simulink model "BasicPumpPlant"  (R2022b)
settings: Solver=VariableStepAuto  StartTime=0.0  StopTime=10.0  RelTol=1e-3
values from neighbouring files (symbols this model uses):
  AN403992StandardFlowMotorMaxDisp_ccperrev = 9.8*2.1    (= 20.58)    [Cascade_SolutionPumpModel_DD.m]
  MotorPumpDampingCoef = 2.630416384778607e-04    (= 0.000263041638478)    [Cascade_SolutionPumpModel_DD.m]
  Pascal_To_psi = 0.0001450377    [Cascade_SolutionPumpModel_DD.m]
undefined symbols (not defined in the file or in its folder): AN402280HighFlowPumpBrakePowerNQ2D_HP, AN403993HighFlowMotorMaxDisp_ccperrev
libraries: fl_lib x21, nesl_utility x9, sh_lib x8, fl_ps_legacy_lib x6, slpidlib x1
settings Model: Creator=pm16590  LastModifiedBy=tilog
settings DataIOCC: ReturnWorkspaceOutputs=off
settings DebuggingCC: UnconnectedInputMsg=warning  UnconnectedOutputMsg=warning  UnconnectedLineMsg=warning  SFMachineParentedDataDiag=warning  ArithmeticOperatorsInVariantConditions=warning
settings ModelReferenceCC: EnableRefExpFcnMdlSchedulingChecks=on
settings SFSimCC: CustomCodeUndefinedFunction=UseInterfaceOnly

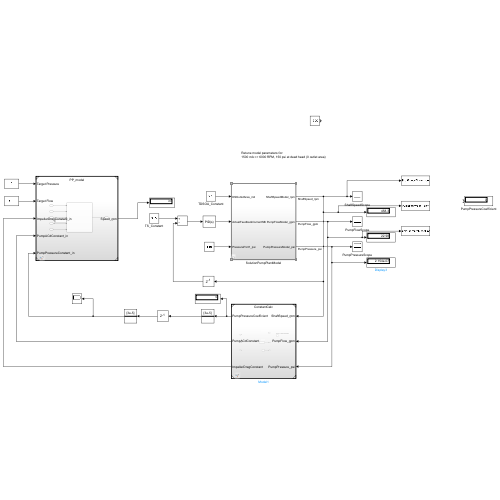
[thumbnail: Simulink's stored preview of the top-level diagram]
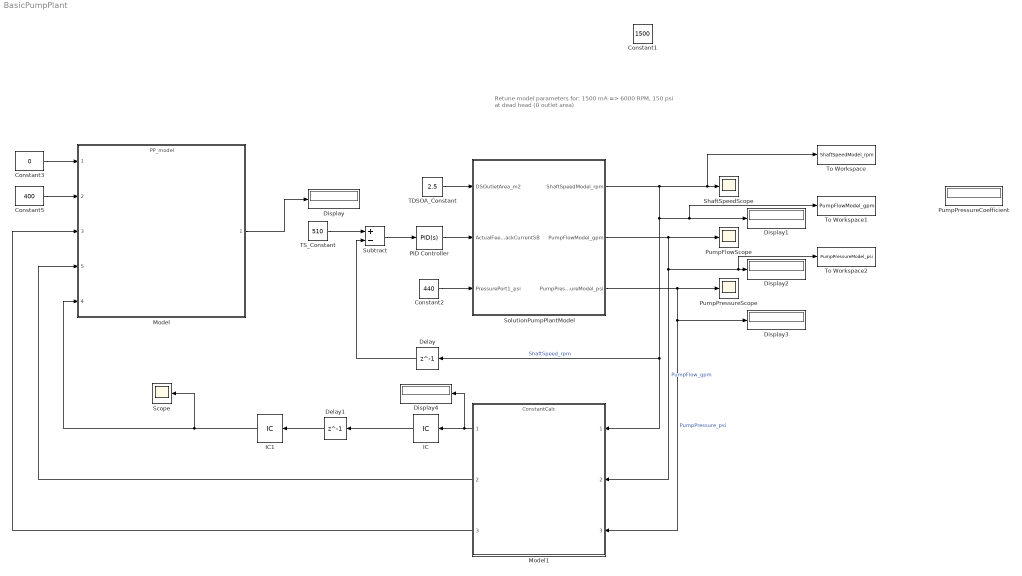
== system BasicPumpPlant ==
  note: Retune model parameters for:
      | 1500 mA => 6000 RPM, 150 psi at dead head (0 outlet area)
  Constant1 : Constant  Value=1500
  Constant2 : Constant  Value=440
  Constant3 : Constant  Value=0
  Constant5 : Constant  Value=400
  Delay : Delay  DelayLength=1  InitialCondition=1
  Delay1 : Delay  DelayLength=1  InitialCondition=1
  Display{,1..4} (5 alike) : Display
  IC : InitialCondition  Value=3e-5
  IC1 : InitialCondition  Value=3e-5
  Model : ModelReference  ModelNameDialog=PP_model.slx  SimulationMode=Normal  ModelReferenceVersion=1.5
      settings: PortSchema="{\"entries\":[{\"content\":{\"sides\":[{\"content\":{\"connectorIds\":[\"In1\",\"In2\",\"In3\",\"In5\",\"In4\"]},\"type\":\"ConnectorPlacement.EquallySpacedRectSide\",\"uuid\":\"fdcef34a-74c4-4aee-b0bc-6e3e5f9e7ac2\"},{\"content\":{\"connectorIds\":[\"Out1\"],\"side\":\"RIGHT\"},\"type\":\"ConnectorPlacement.EquallySpacedRectSide\",\"uuid\":\"cb4b70af-0550-4c5a-8289-d3aa2bf45742\"},{\"content\":{\"connectorIds\":[],\"side\":\"TOP\"},\"type\":\"ConnectorPlacement.EquallySpacedRectSide\",\"uuid\":\"87759187-0da6-406f-b9db-6c95d92bffe7\"}]},\"type\":\"ConnectorPlacement.EquallySpacedConnector\",\"uuid\":\"123e04ed-575d-4795-8cdc-174c34b6de50\"}],\"packageUris\":[\"http://schema.mathworks.com/mf0/Connector/R2020b\"],\"version\":\"1.0\"}"
  Model1 : ModelReference  ModelNameDialog=ConstantCalc.slx  SimulationMode=Normal  ModelReferenceVersion=1.11
  PID Controller : slpidlib/PID Controller  Controller=PID  Form=Parallel  TimeDomain=Continuous-time  UseExternalTs=off  SampleTime=-1  IntegratorMethod=Forward Euler  FilterMethod=Forward Euler  ControllerParametersSource=internal  P=0  I=.1  UseKiTs=off  D=0  N=100  UseFilter=on  TunerSelectOption=Transfer Function Based (PID Tuner App)  InitialConditionSource=internal  InitialConditionForIntegrator=0  InitialConditionForFilter=0  DifferentiatorICPrevScaledInput=0  ExternalReset=none  TrackingMode=off  Kt=1  LimitOutput=off  SatLimitsSource=internal  UpperSaturationLimit=inf  LowerSaturationLimit=-inf  LinearizeAsGain=on  AntiWindupMode=none  Kb=1  LimitIntegrator=off  UpperIntegratorSaturationLimit=inf  LowerIntegratorSaturationLimit=-inf  POutMin=[]  POutMax=[]  IOutMin=[]  IOutMax=[]  DOutMin=[]  DOutMax=[]  NOutMin=[]  NOutMax=[]  SumOutMin=[]  SumOutMax=[]  SaturationOutMin=[]  SaturationOutMax=[]  PParamMin=[]  PParamMax=[]  IParamMin=[]  IParamMax=[]  DParamMin=[]  DParamMax=[]  NParamMin=[]  NParamMax=[]  KbParamMin=[]  KbParamMax=[]  KtParamMin=[]  KtParamMax=[]  KbOutMin=[]  KbOutMax=[]  KtOutMin=[]  KtOutMax=[]  IntegratorOutMin=[]  IntegratorOutMax=[]  FilterOutMin=[]  FilterOutMax=[]  SumI1OutMin=[]  SumI1OutMax=[]  SumI2OutMin=[]  SumI2OutMax=[]  SumI3OutMin=[]  SumI3OutMax=[]  SumI4OutMin=[]  SumI4OutMax=[]  SumDOutMin=[]  SumDOutMax=[]  DifferentiatorOutMin=[]  DifferentiatorOutMax=[]  FilterDiffOutCoefMin=[]  FilterDiffOutCoefMax=[]  ReciprocalOutMin=[]  ReciprocalOutMax=[]  SumDenOutMin=[]  SumDenOutMax=[]  SumNumOutMin=[]  SumNumOutMax=[]  DivideOutMin=[]  DivideOutMax=[]  UdiffTsProdOutMin=[]  UdiffTsProdOutMax=[]  NTsProdOutMin=[]  NTsProdOutMax=[]  UintegralTsProdOutMin=[]  UintegralTsProdOutMax=[]  UngainTsProdOutMin=[]  UngainTsProdOutMax=[]  ClampingZeroOutDataTypeStr=Inherit: Inherit via back propagation  ClampingZeroOutMin=[]  ClampingZeroOutMax=[]  FilterDenConstantOutDataTypeStr=Inherit: Inherit via back propagation  FilterDenConstantOutMin=[]  FilterDenConstantOutMax=[]  PCopyOutDataTypeStr=Inherit: Inherit via back propagation  PCopyOutMin=[]  PCopyOutMax=[]  NCopyOutDataTypeStr=Inherit: Inherit via back propagation  NCopyOutMin=[]  NCopyOutMax=[]  IntegratorContinuousStateAttributes=''  IntegratorStateMustResolveToSignalObject=off  IntegratorRTWStateStorageClass=Auto  FilterContinuousStateAttributes=''  FilterStateMustResolveToSignalObject=off  FilterRTWStateStorageClass=Auto  ParallelPVariant=InternalParameters  IdealPVariant=Disabled  IVariant=InternalParameters  DVariant=InternalParameters  IntegratorVariant=Continuous  SatVariant=Disabled  AWVariant=Passthrough  PCopyVariant=Disabled  TRVariant=Disabled  FdbkBlocksVariant=Forward  IdealPFdbkVariant=Disabled  SatFdbkVariant=Disabled  DerivativeFilterVariant=ContFilter  NVariant=InternalParameters  NCopyVariant=Disabled  FilterICVariant=InternalICsFilter  IntegratorICVariant=InternalICs  ExternalResetVariant=Disabled  TRSumVariant=Passthrough  SumFdbkVariant=Disabled  SumVariant=Sum_PID  TsampFilterVariant=InternalTs  TsampNgainVariant=Passthrough  TsampIntegralVariant=Passthrough  ExternalSaturationOutDataTypeStr=Inherit: Same as second input
  PumpFlowScope : Scope
  PumpPressureCoefficient : Display
  PumpPressureScope : Scope
  Scope : Scope
  ShaftSpeedScope : Scope
  SolutionPumpPlantModel : Subsystem  AncestorBlock=Cascade_SolutionSystemPumpModel_Library/MIL1/PlantModel/MIL1  StartFcn=|  StopFcn=|
      StartFcn=|
      | try
      |   JD_ModelUsageLogCallback('start','Plant');
      | end
      StopFcn=|
      | try
      |   JD_ModelUsageLogCallback('stop','Plant');
      | end
      settings: LibrarySourceBlock=Cascade_SolutionSystemPumpModel_Library/MIL1/PlantModel/MIL1
  Subtract : Sum  Inputs=+-
  TDSOA_Constant : Constant  Value=2.5
  TS_Constant : Constant  Value=510
  To Workspace : ToWorkspace  VariableName=ShaftSpeedModel_rpm  SaveFormat=Structure With Time  SampleTime=-1
  To Workspace1 : ToWorkspace  VariableName=PumpFlowModel_gpm  SaveFormat=Structure With Time  SampleTime=-1
  To Workspace2 : ToWorkspace  VariableName=PumpPressureModel_psi  SaveFormat=Structure With Time  SampleTime=-1
  wires:
  TDSOA_Constant/1 -> SolutionPumpPlantModel/1(DSOutletArea_m2)
  SolutionPumpPlantModel/1(ShaftSpeedModel_rpm) -> To Workspace/1, ShaftSpeedScope/1, Display1/1, To Workspace1/1, Model1/1, Delay/1  "ShaftSpeed_rpm"
  SolutionPumpPlantModel/2(PumpFlowModel_gpm) -> Model1/2, To Workspace2/1, Display2/1, PumpFlowScope/1  "PumpFlow_gpm"
  SolutionPumpPlantModel/3(PumpPressureModel_psi) -> PumpPressureScope/1, Model1/3, Display3/1  "PumpPressure_psi"
  Constant2/1 -> SolutionPumpPlantModel/3(PressurePort1_psi)
  Constant3/1 -> Model/1
  Constant5/1 -> Model/2
  PID Controller/1 -> SolutionPumpPlantModel/2(ActualFeedbackCurrentSB)
  Subtract/1 -> PID Controller/1
  Model/1 -> Display/1
  Delay/1 -> Subtract/2
  Model1/2 -> Model/5
  Model1/3 -> Model/3
  Model1/1 -> Display4/1, IC/1
  Delay1/1 -> IC1/1
  IC/1 -> Delay1/1
  IC1/1 -> Scope/1, Model/4
  TS_Constant/1 -> Subtract/1

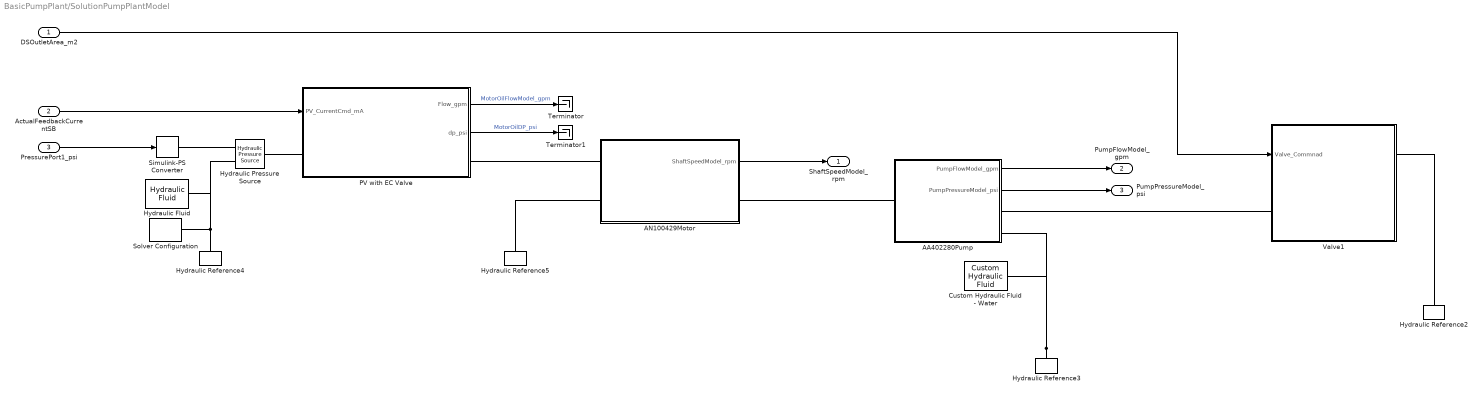
== system BasicPumpPlant/SolutionPumpPlantModel ==
  DSOutletArea_m2 : Inport
  ActualFeedbackCurrentSB : Inport  Port=2
  PressurePort1_psi : Inport  Port=3
  AA402280Pump : Subsystem
      mask Display: image('Pump.png')
  AN100429Motor : Subsystem
      mask Display: image('motor.png')
  Custom Hydraulic Fluid - Water : fl_lib/Hydraulic/Hydraulic Utilities/Custom Hydraulic Fluid  density=Fluid_density_kgm3 kg/m^3  viscosity_kin=Viscocity_cSt cSt  bulk=Bulk_Modulus_Pa Pa  alpha=Trapped_air  range_error=2
      settings: InternalSimscapePortConfiguration="{\"Bottom\":[],\"Left\":[],\"Right\":[{\"id\":\"G\",\"label\":\"\",\"type\":\"foundation.hydraulic.hydraulic\"}],\"Top\":[]}"
  Hydraulic Fluid : sh_lib/Hydraulic Utilities/Hydraulic Fluid  SelFluid=9  SysTemp=25  TrapAir=0.005  ViscDerFactor=1  range_error=2
  Hydraulic Pressure Source : fl_lib/Hydraulic/Hydraulic Sources/Hydraulic Pressure Source
      settings: InternalSimscapePortConfiguration="{\"Bottom\":[],\"Left\":[{\"id\":\"P\",\"label\":\"P\",\"type\":\"foundation.hydraulic.hydraulic\"}],\"Right\":[{\"id\":\"S\",\"label\":\"S\",\"type\":\"input\"},{\"id\":\"T\",\"label\":\"T\",\"type\":\"foundation.hydraulic.hydraulic\"}],\"Top\":[]}"
  Hydraulic Reference{2..5} (4 alike) : fl_lib/Hydraulic/Hydraulic Elements/Hydraulic Reference
  PV with EC Valve : Subsystem
  Simulink-PS Converter : nesl_utility/Simulink-PS Converter  PhysicalDomain=network_engine_domain  SubClassName=ps_input  LeftPortType=input  RightPortType=output  PseudoPeriodic=off  Frequencies=[]  NoiseDistribution=none  NoiseParameters=[]  Unit=psi  AffineConversion=off  FilteringAndDerivatives=zero  SimscapeFilterOrder=1  InputFilterTimeConstant=0.001  UdotUserProvided=0
  Solver Configuration : nesl_utility/Solver Configuration  PhysicalDomain=network_engine_domain  SubClassName=solver  LeftPortType=input  RightPortType=generic  Tones=[]  Harmonics=[]  SimulateNoise=off  Profile=off  UseLocalSampling=off  EnableSwitchedLinearOptims=on  FrequencyDomain=off  UseCCode=off  RelTol=0.001  AbsTol=1e-06  MinStep=1e-09  ToWorkspace=off  RevertToSquareIcSolve=off  NumHomotopyIterations=100  PhasorMode=off  PhasorModeNumHarmonics=1  ConsistencySolver=NEWTON_FTOL  IndexReductionMethod=DerivativeReplacement  DoDC=off  ResidualTolerance=1e-9  ConsistencyTolSource=GLOBAL  ConsistencyAbsTol=0.001  ConsistencyRelTol=0.001  ConsistencyTolFactor=0.001  UseLocalSolver=off  LocalSolverChoice=NE_BACKWARD_EULER_ADVANCER  ResolveIndetEquations=on  FunctionEvalNumThread=1  LocalSolverSampleTime=0.001  DoFixedCost=off  MaxNonlinIter=3  MaxModeIter=2  ComputeImpulses=off  ImpulseIterations=2  LinearAlgebra=Sparse  LinearAlgebraNumThread=0  EquationFormulation=NE_TIME_EF  DelaysMemoryBudget=1024  AutomaticFiltering=off  FilteringTimeConstant=0.01  PartitionStorageMethod=AS_NEEDED  PartitionMemoryBudget=1024  PartitionMethod=FAST
  Terminator : Terminator
  Terminator1 : Terminator
  Valve1 : Subsystem
      mask Display: image('Variable_Orifice.png')
  ShaftSpeedModel_rpm : Outport  VectorParamsAs1DForOutWhenUnconnected=off
  PumpFlowModel_gpm : Outport  Port=2  VectorParamsAs1DForOutWhenUnconnected=off
  PumpPressureModel_psi : Outport  Port=3  VectorParamsAs1DForOutWhenUnconnected=off
  wires:
  DSOutletArea_m2/1 -> Valve1/1(Valve_Commnad)
  AA402280Pump/1(PumpFlowModel_gpm) -> PumpFlowModel_gpm/1
  AA402280Pump/2(PumpPressureModel_psi) -> PumpPressureModel_psi/1
  AN100429Motor/1(ShaftSpeedModel_rpm) -> ShaftSpeedModel_rpm/1
  PV with EC Valve/1(Flow_gpm) -> Terminator/1  "MotorOilFlowModel_gpm"
  ActualFeedbackCurrentSB/1 -> PV with EC Valve/1(PV_CurrentCmd_mA)
  PV with EC Valve/2(dp_psi) -> Terminator1/1  "MotorOilDP_psi"
  PressurePort1_psi/1 -> Simulink-PS Converter/1
  connections:
  AN100429Motor/LConn2 -- Hydraulic Reference5/LConn1
  PV with EC Valve/RConn1 -- AN100429Motor/LConn1
  AA402280Pump/LConn1 -- AN100429Motor/RConn1
  Hydraulic Reference2/LConn1 -- Valve1/RConn1
  Valve1/LConn1 -- AA402280Pump/RConn1
  PV with EC Valve/LConn1 -- Hydraulic Pressure Source/LConn1
  Simulink-PS Converter/RConn1 -- Hydraulic Pressure Source/RConn1
  Hydraulic Reference4/LConn1 -- Solver Configuration/RConn1 -- Hydraulic Fluid/RConn1 -- Hydraulic Pressure Source/RConn2
  Hydraulic Reference3/LConn1 -- Custom Hydraulic Fluid - Water/RConn1 -- AA402280Pump/RConn2

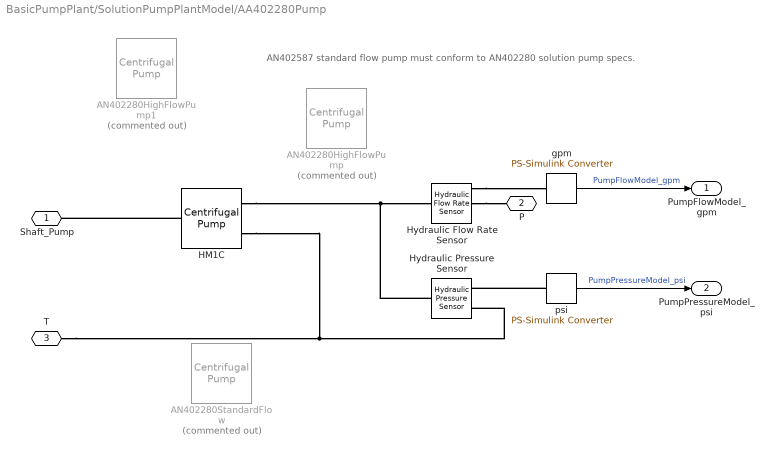
== system BasicPumpPlant/SolutionPumpPlantModel/AA402280Pump ==
  note: AN402587 standard flow pump must conform to AN402280 solution pump specs.
  AN402280HighFlowPump : sh_lib/Pumps and Motors/Centrifugal Pump  Commented=on  mdl_type=2  c_1=326.8 Pa/(kg/m^3)  c_2=3.104e+4 Pa*s/kg  c_3=1.097e+7 Pa*s^2/(kg*m^3)  c_4=2.136e+5 Pa*s^2/(kg*m^3)  c_f=0.8  design_del=130 lpm  ref_velocity=AN402280HighFlowPumpRefVelocity_rpm rpm  ref_density=AN402280HighFlowPumpRefDensity_kgperm3 kg/m^3  leak_resistance=1e+8 Pa/(m^3/s)  T_const=0.1 N*m  trq_press_coeff=1e-6 N*m/Pa  pump_del_1D=AN402280HighFlowPumpDelievery_gpm gpm  press_diff_1D=AN402280HighFlowPDiff_psi psi  pump_del_power_1D=AN402280HighFlowPumpDelievery_gpm gpm  power_1D=AN402280HighFlowPumpBrakePowerNQ_HP HP  pump_vel_2D=[ 3.2e+3 3.3e+3 3.4e+3 3.5e+3 ] rpm  pump_del_2D=[ 0 50 100 150 200 250 300 350 ] lpm  press_diff_2D=[ 8.300000000000001 8.800000000000001 9.300000000000001 9.9; 7.8 8.300000000000001 8.800000000000001 9.4; 7.2 7.6 8.199999999999999 8.699999999999999; 6.5 7 7.5 8; 5.6 6.1 6.6 7.1; 4.7 5.2 5.7 6.2; 3.4 4 4.4 4.9; 2.3 2.7 3.4 3.6 ] bar  pump_del_power_2D=[ 0 50 100 150 200 250 300 350 ] lpm  power_2D=[ 1.223e+3 1.341e+3 1.467e+3 1.6e+3; 1.414e+3 1.551e+3 1.696e+3 1.85e+3; 1.636e+3 1.794e+3 1.962e+3 2.14e+3; 1.941e+3 2.129e+3 2.326e+3 2.54e+3; 2.224e+3 2.439e+3 2.66e+3 2.91e+3; 2.453e+3 2.691e+3 2.947e+3 3.21e+3; 2.757e+3 3.024e+3 3.307e+3 3.608e+3; 2.945e+3 3.23e+3 3.533e+3 3.854e+3 ] W  omega_threshold=1e-9 rad/s  interp_method=1  extrap_method=1
      settings: InternalSimscapePortConfiguration="{\"Bottom\":[],\"Left\":[{\"id\":\"S\",\"label\":\"S\",\"type\":\"foundation.mechanical.rotational.rotational\"}],\"Right\":[{\"id\":\"P\",\"label\":\"P\",\"type\":\"foundation.hydraulic.hydraulic\"},{\"id\":\"T\",\"label\":\"T\",\"type\":\"foundation.hydraulic.hydraulic\"}],\"Top\":[]}"
  AN402280HighFlowPump1 : sh_lib/Pumps and Motors/Centrifugal Pump  Commented=on  mdl_type=3  c_1=326.8 Pa/(kg/m^3)  c_2=3.104e+4 Pa*s/kg  c_3=1.097e+7 Pa*s^2/(kg*m^3)  c_4=2.136e+5 Pa*s^2/(kg*m^3)  c_f=0.8  design_del=130 lpm  ref_velocity=AN402280HighFlowPumpRefVelocity_rpm rpm  ref_density=AN402280HighFlowPumpRefDensity_kgperm3 kg/m^3  leak_resistance=1e+8 Pa/(m^3/s)  T_const=0.1 N*m  trq_press_coeff=1e-6 N*m/Pa  pump_del_1D=AN402280HighFlowPumpDelievery_gpm gpm  press_diff_1D=AN402280HighFlowPDiff_psi psi  pump_del_power_1D=AN402280HighFlowPumpDelievery_gpm gpm  power_1D=AN402280HighFlowPumpBrakePowerNQ_HP HP  pump_vel_2D=AN402280HighFlowAngulerVelocity2D_rpm rpm  pump_del_2D=AN402280HighFlowPumpDelievery_gpm gpm  press_diff_2D=AN402280HighFlowPDiff2D_psi psi  pump_del_power_2D=AN402280HighFlowPumpDelievery_gpm gpm  power_2D=AN402280HighFlowPumpBrakePowerNQ2D_HP' HP  omega_threshold=1e-9 rad/s  interp_method=1  extrap_method=1
      settings: InternalSimscapePortConfiguration="{\"Bottom\":[],\"Left\":[{\"id\":\"S\",\"label\":\"S\",\"type\":\"foundation.mechanical.rotational.rotational\"}],\"Right\":[{\"id\":\"P\",\"label\":\"P\",\"type\":\"foundation.hydraulic.hydraulic\"},{\"id\":\"T\",\"label\":\"T\",\"type\":\"foundation.hydraulic.hydraulic\"}],\"Top\":[]}"
  AN402280StandardFlow : sh_lib/Pumps and Motors/Centrifugal Pump  Commented=on  mdl_type=2  c_1=326.8 Pa/(kg/m^3)  c_2=3.104e+4 Pa*s/kg  c_3=1.097e+7 Pa*s^2/(kg*m^3)  c_4=2.136e+5 Pa*s^2/(kg*m^3)  c_f=0.8  design_del=130 lpm  ref_velocity=AN402280StdFlowPumpRefVelocity_rpm rpm  ref_density=AN402280StdFlowPumpRefDensity_kgperm3 kg/m^3  leak_resistance=1e+8 Pa/(m^3/s)  T_const=0.1 N*m  trq_press_coeff=1e-6 N*m/Pa  pump_del_1D=AN402280StdFlowPumpDelievery_gpm gpm  press_diff_1D=AN402280StdFlowPDiff_psi psi  pump_del_power_1D=AN402280StdFlowPumpDelievery_gpm gpm  power_1D=AN402280StdFlowPumpBrakePowerNQ_HP HP  pump_vel_2D=[ 3.2e+3 3.3e+3 3.4e+3 3.5e+3 ] rpm  pump_del_2D=[ 0 50 100 150 200 250 300 350 ] lpm  press_diff_2D=[ 8.300000000000001 8.800000000000001 9.300000000000001 9.9; 7.8 8.300000000000001 8.800000000000001 9.4; 7.2 7.6 8.199999999999999 8.699999999999999; 6.5 7 7.5 8; 5.6 6.1 6.6 7.1; 4.7 5.2 5.7 6.2; 3.4 4 4.4 4.9; 2.3 2.7 3.4 3.6 ] bar  pump_del_power_2D=[ 0 50 100 150 200 250 300 350 ] lpm  power_2D=[ 1.223e+3 1.341e+3 1.467e+3 1.6e+3; 1.414e+3 1.551e+3 1.696e+3 1.85e+3; 1.636e+3 1.794e+3 1.962e+3 2.14e+3; 1.941e+3 2.129e+3 2.326e+3 2.54e+3; 2.224e+3 2.439e+3 2.66e+3 2.91e+3; 2.453e+3 2.691e+3 2.947e+3 3.21e+3; 2.757e+3 3.024e+3 3.307e+3 3.608e+3; 2.945e+3 3.23e+3 3.533e+3 3.854e+3 ] W  omega_threshold=1e-9 rad/s  interp_method=1  extrap_method=1
      settings: InternalSimscapePortConfiguration="{\"Bottom\":[],\"Left\":[{\"id\":\"S\",\"label\":\"S\",\"type\":\"foundation.mechanical.rotational.rotational\"}],\"Right\":[{\"id\":\"P\",\"label\":\"P\",\"type\":\"foundation.hydraulic.hydraulic\"},{\"id\":\"T\",\"label\":\"T\",\"type\":\"foundation.hydraulic.hydraulic\"}],\"Top\":[]}"
  HM1C : sh_lib/Pumps and Motors/Centrifugal Pump  mdl_type=2  c_1=326.8 Pa/(kg/m^3)  c_2=3.104e+4 Pa*s/kg  c_3=1.097e+7 Pa*s^2/(kg*m^3)  c_4=2.136e+5 Pa*s^2/(kg*m^3)  c_f=0.8  design_del=130 lpm  ref_velocity=HM1CPumpRefVelocity_rpm rpm  ref_density=HM1CPumpRefDensity_kgperm3 kg/m^3  leak_resistance=1e+8 Pa/(m^3/s)  T_const=0.1 N*m  trq_press_coeff=1e-6 N*m/Pa  pump_del_1D=HM1CPumpDelievery_gpm gpm  press_diff_1D=HM1CPumpPDiff_psi psi  pump_del_power_1D=HM1CPumpDelievery_gpm gpm  power_1D=HM1CPumpBrakePowerNQ_HP HP  pump_vel_2D=0 rpm  pump_del_2D=0 gpm  press_diff_2D=0 psi  pump_del_power_2D=0 gpm  power_2D=0 HP  omega_threshold=1e-9 rad/s  interp_method=1  extrap_method=1
      settings: InternalSimscapePortConfiguration="{\"Bottom\":[],\"Left\":[{\"id\":\"S\",\"label\":\"S\",\"type\":\"foundation.mechanical.rotational.rotational\"}],\"Right\":[{\"id\":\"P\",\"label\":\"P\",\"type\":\"foundation.hydraulic.hydraulic\"},{\"id\":\"T\",\"label\":\"T\",\"type\":\"foundation.hydraulic.hydraulic\"}],\"Top\":[]}"
  Hydraulic Flow Rate Sensor : fl_lib/Hydraulic/Hydraulic Sensors/Hydraulic Flow Rate Sensor
  Hydraulic Pressure Sensor : fl_lib/Hydraulic/Hydraulic Sensors/Hydraulic Pressure Sensor
  gpm : nesl_utility/PS-Simulink Converter  PhysicalDomain=network_engine_domain  SubClassName=ps_output  LeftPortType=input  RightPortType=output  PseudoPeriodic=off  Frequencies=[]  VectorFormat=1-D array  Unit=gpm  AffineConversion=off
  psi : nesl_utility/PS-Simulink Converter  PhysicalDomain=network_engine_domain  SubClassName=ps_output  LeftPortType=input  RightPortType=output  PseudoPeriodic=off  Frequencies=[]  VectorFormat=1-D array  Unit=psi  AffineConversion=off
  Shaft_Pump : PMIOPort  Side=Left
  P : PMIOPort  Port=2  Side=Right
  T : PMIOPort  Port=3  Side=Right
  PumpFlowModel_gpm : Outport  VectorParamsAs1DForOutWhenUnconnected=off
  PumpPressureModel_psi : Outport  Port=2  VectorParamsAs1DForOutWhenUnconnected=off
  wires:
  psi/1 -> PumpPressureModel_psi/1  "PumpPressureModel_psi"
  gpm/1 -> PumpFlowModel_gpm/1  "PumpFlowModel_gpm"
  connections:
  psi/LConn1 -- Hydraulic Pressure Sensor/RConn2
  Hydraulic Flow Rate Sensor/RConn1 -- gpm/LConn1
  Hydraulic Flow Rate Sensor/RConn2 -- P/RConn1
  HM1C/LConn1 -- Shaft_Pump/RConn1
  HM1C/RConn2 -- Hydraulic Pressure Sensor/RConn1 -- T/RConn1
  HM1C/RConn1 -- Hydraulic Flow Rate Sensor/LConn1 -- Hydraulic Pressure Sensor/LConn1

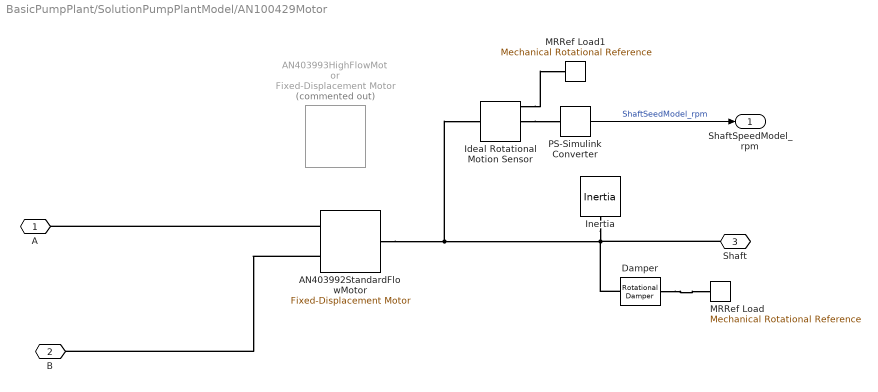
== system BasicPumpPlant/SolutionPumpPlantModel/AN100429Motor ==
  AN403992StandardFlowMotor : sh_lib/Pumps and Motors/Fixed-Displacement Motor  D="AN403992StandardFlowMotorMaxDisp_ccperrev  cm^3/rev"  loss_spec=1  w_nominal=AN403992StandardFlowMotorRatedSpeed_rpm rpm  pr_nominal=MotorNominalDelP_pa Pa  visc_nominal=34.92 cSt  dens_nominal=840 kg/m^3  efficiency_vol=MotorHydOilVolEff  no_load_torque=0.5 N*m  torque_pressure_coeff=0 N*m/Pa  p_diff_eff_TLU=[100000, 1000000, 2000000] Pa  omega_eff_TLU=[25, 50, 100, 200, 300, 400] rad/s  vol_eff_TLU=[.816, .908, .954, .977, .981, .984; .325, .663, .831, .916, .925, .946; .137, .568, .78, .892, .893, .91]  mech_eff_TLU=[.996, .996, .996, .996, .996, .996; .988, .989, .989, .989, .989, .99; .981, .981, .982, .982, .983, .984]  p_diff_loss_TLU=[100000, 1000000, 2000000] Pa  omega_loss_TLU=[25, 50, 100, 200, 300, 400] rad/s  vol_loss_TLU=[.0282, .0253, .0241, .0235, .0291, .0325; .2596, .1271, .1017, .0917, .1216, .1142; .7874, .1901, .141, .1211, .1797, .1978] * 1e-3 m^3/s  mech_loss_TLU=[.002, .002, .002, .002, .002, .002; .06, .055, .055, .055, .055, .05; .19, .19, .18, .18, .17, .16] N*m  pressure_threshold=1e5 Pa  omega_threshold=10 rad/s  quadrant_check=0  pressure_check=0  min_valid_pressure=0 Pa  vol_eff_min=1e-3  vol_eff_max=1  mech_eff_min=1e-3  mech_eff_max=1
      settings: InternalSimscapePortConfiguration="{\"Bottom\":[],\"Left\":[{\"id\":\"A\",\"label\":\"A\",\"type\":\"foundation.hydraulic.hydraulic\"},{\"id\":\"B\",\"label\":\"B\",\"type\":\"foundation.hydraulic.hydraulic\"}],\"Right\":[{\"id\":\"S\",\"label\":\"S\",\"type\":\"foundation.mechanical.rotational.rotational\"}],\"Top\":[]}"
  AN403993HighFlowMotor : sh_lib/Pumps and Motors/Fixed-Displacement Motor  Commented=on  D=AN403993HighFlowMotorMaxDisp_ccperrev cm^3/rev  loss_spec=1  w_nominal=AN403993HighFlowMotorRatedSpeed_rpm rpm  pr_nominal=MotorNominalDelP_pa Pa  visc_nominal=34.92 cSt  dens_nominal=840 kg/m^3  efficiency_vol=MotorHydOilVolEff  no_load_torque=0.5 N*m  torque_pressure_coeff=0 N*m/Pa  p_diff_eff_TLU=[100000, 1000000, 2000000] Pa  omega_eff_TLU=[25, 50, 100, 200, 300, 400] rad/s  vol_eff_TLU=[.816, .908, .954, .977, .981, .984; .325, .663, .831, .916, .925, .946; .137, .568, .78, .892, .893, .91]  mech_eff_TLU=[.996, .996, .996, .996, .996, .996; .988, .989, .989, .989, .989, .99; .981, .981, .982, .982, .983, .984]  p_diff_loss_TLU=[100000, 1000000, 2000000] Pa  omega_loss_TLU=[25, 50, 100, 200, 300, 400] rad/s  vol_loss_TLU=[.0282, .0253, .0241, .0235, .0291, .0325; .2596, .1271, .1017, .0917, .1216, .1142; .7874, .1901, .141, .1211, .1797, .1978] * 1e-3 m^3/s  mech_loss_TLU=[.002, .002, .002, .002, .002, .002; .06, .055, .055, .055, .055, .05; .19, .19, .18, .18, .17, .16] N*m  pressure_threshold=1e5 Pa  omega_threshold=10 rad/s  quadrant_check=0  pressure_check=0  min_valid_pressure=0 Pa  vol_eff_min=1e-3  vol_eff_max=1  mech_eff_min=1e-3  mech_eff_max=1
      settings: InternalSimscapePortConfiguration="{\"Bottom\":[],\"Left\":[{\"id\":\"A\",\"label\":\"A\",\"type\":\"foundation.hydraulic.hydraulic\"},{\"id\":\"B\",\"label\":\"B\",\"type\":\"foundation.hydraulic.hydraulic\"}],\"Right\":[{\"id\":\"S\",\"label\":\"S\",\"type\":\"foundation.mechanical.rotational.rotational\"}],\"Top\":[]}"
  Damper : fl_lib/Mechanical/Rotational Elements/Rotational Damper  Tag=Factory Generic  D=MotorPumpDampingCoef N*m/(rad/s)  w_specify=off  w_priority=High  w=0 rad/s  w_nominal_specify=off  w_nominal_unit=rad/s  w_nominal_value=1  t_specify=off  t_priority=High  t=0 N*m  t_nominal_specify=off  t_nominal_unit=N*m  t_nominal_value=1
  Ideal Rotational Motion Sensor : fl_lib/Mechanical/Mechanical Sensors/Ideal Rotational Motion Sensor  reference=foundation.enum.MeasurementReference.difference  acceleration_port=false  velocity_port=true  position_port=true  wrap_angle=false  offset=0 rad
  Inertia : fl_lib/Mechanical/Rotational Elements/Inertia  Tag=Factory Generic  inertia=MotorPumpInertia_kgm2 kg*m^2  num_ports=foundation.enum.numPorts2.one  w_specify=on  w_priority=High  w=0 rad/s  w_nominal_specify=off  w_nominal_unit=rad/s  w_nominal_value=1  t_specify=off  t_priority=High  t=0 N*m  t_nominal_specify=off  t_nominal_unit=N*m  t_nominal_value=1
  MRRef Load : fl_lib/Mechanical/Rotational Elements/Mechanical Rotational Reference  Tag=Factory Generic
  MRRef Load1 : fl_lib/Mechanical/Rotational Elements/Mechanical Rotational Reference  Tag=Factory Generic
  PS-Simulink Converter : nesl_utility/PS-Simulink Converter  PhysicalDomain=network_engine_domain  SubClassName=ps_output  LeftPortType=input  RightPortType=output  PseudoPeriodic=off  Frequencies=[]  VectorFormat=1-D array  Unit=rpm  AffineConversion=off
  A : PMIOPort  Side=Left
  B : PMIOPort  Port=2  Side=Left
  Shaft : PMIOPort  Port=3  Side=Right
  ShaftSpeedModel_rpm : Outport  VectorParamsAs1DForOutWhenUnconnected=off
  wires:
  PS-Simulink Converter/1 -> ShaftSpeedModel_rpm/1  "ShaftSeedModel_rpm"
  connections:
  Shaft/RConn1 -- Damper/LConn1 -- Ideal Rotational Motion Sensor/LConn1 -- AN403992StandardFlowMotor/RConn1 -- Inertia/LConn1
  Ideal Rotational Motion Sensor/RConn1 -- MRRef Load1/LConn1
  AN403992StandardFlowMotor/LConn2 -- B/RConn1
  Damper/RConn1 -- MRRef Load/LConn1
  Ideal Rotational Motion Sensor/RConn2 -- PS-Simulink Converter/LConn1
  AN403992StandardFlowMotor/LConn1 -- A/RConn1

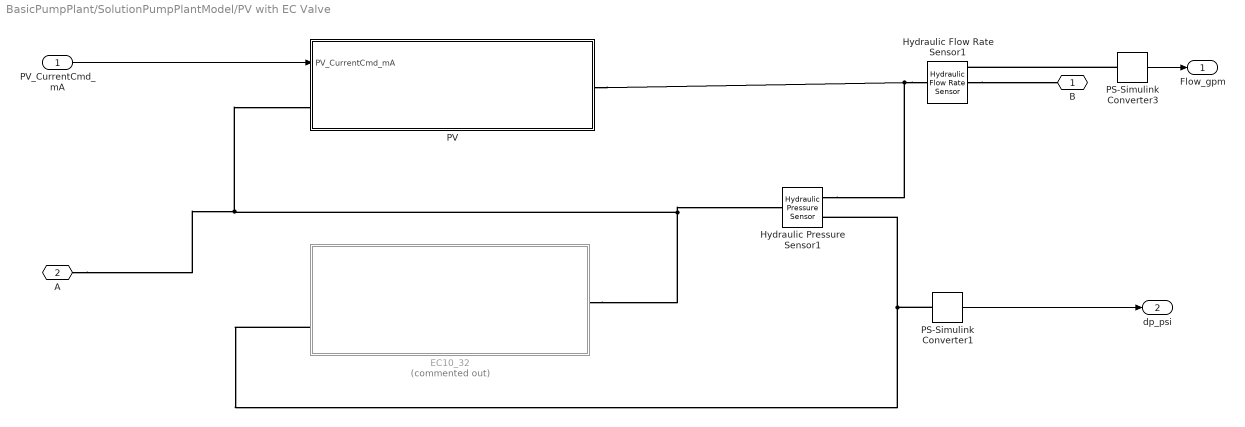
== system BasicPumpPlant/SolutionPumpPlantModel/PV with EC Valve ==
  PV_CurrentCmd_mA : Inport
  EC10_32 : Subsystem  Commented=on
  Hydraulic Flow Rate Sensor1 : fl_lib/Hydraulic/Hydraulic Sensors/Hydraulic Flow Rate Sensor
  Hydraulic Pressure Sensor1 : fl_lib/Hydraulic/Hydraulic Sensors/Hydraulic Pressure Sensor
  PS-Simulink Converter1 : nesl_utility/PS-Simulink Converter  PhysicalDomain=network_engine_domain  SubClassName=ps_output  LeftPortType=input  RightPortType=output  PseudoPeriodic=off  Frequencies=[]  VectorFormat=1-D array  Unit=psi  AffineConversion=off
  PS-Simulink Converter3 : nesl_utility/PS-Simulink Converter  PhysicalDomain=network_engine_domain  SubClassName=ps_output  LeftPortType=input  RightPortType=output  PseudoPeriodic=off  Frequencies=[]  VectorFormat=1-D array  Unit=gpm  AffineConversion=off
  PV : Subsystem
  B : PMIOPort  Side=Right
  A : PMIOPort  Port=2  Side=Left
  Flow_gpm : Outport  VectorParamsAs1DForOutWhenUnconnected=off
  dp_psi : Outport  Port=2  VectorParamsAs1DForOutWhenUnconnected=off
  wires:
  PV_CurrentCmd_mA/1 -> PV/1(PV_CurrentCmd_mA)
  PS-Simulink Converter3/1 -> Flow_gpm/1
  PS-Simulink Converter1/1 -> dp_psi/1
  connections:
  Hydraulic Flow Rate Sensor1/LConn1 -- PV/RConn1 -- Hydraulic Pressure Sensor1/RConn1
  A/RConn1 -- Hydraulic Pressure Sensor1/LConn1 -- EC10_32/RConn1 -- PV/LConn1
  Hydraulic Pressure Sensor1/RConn2 -- EC10_32/LConn2 -- PS-Simulink Converter1/LConn1
  PS-Simulink Converter3/LConn1 -- Hydraulic Flow Rate Sensor1/RConn1
  Hydraulic Flow Rate Sensor1/RConn2 -- B/RConn1

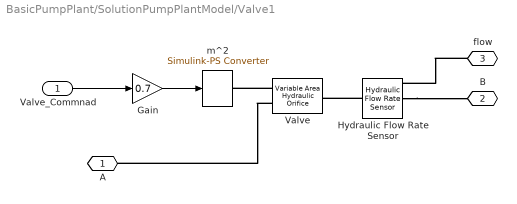
== system BasicPumpPlant/SolutionPumpPlantModel/Valve1 ==
  Valve_Commnad : Inport
  Gain : Gain  Gain=0.7
  Hydraulic Flow Rate Sensor : fl_lib/Hydraulic/Hydraulic Sensors/Hydraulic Flow Rate Sensor
  Valve : fl_lib/Hydraulic/Hydraulic Elements/Variable Area Hydraulic Orifice  C_d=0.6  min_area=1e-15 m^2  lam_spec=2  B_lam=0.999  Re_cr=12  q_specify=off  q_priority=None  q=0 m^3/s  q_nominal_specify=off  q_nominal_unit=m^3/s  q_nominal_value=1  p_specify=off  p_priority=None  p=0 Pa  p_nominal_specify=off  p_nominal_unit=Pa  p_nominal_value=1
      settings: InternalSimscapePortConfiguration="{\"Bottom\":[],\"Left\":[{\"id\":\"AR\",\"label\":\"AR\",\"type\":\"input\"},{\"id\":\"A\",\"label\":\"A\",\"type\":\"foundation.hydraulic.hydraulic\"}],\"Right\":[{\"id\":\"B\",\"label\":\"B\",\"type\":\"foundation.hydraulic.hydraulic\"}],\"Top\":[]}"
  m^2 : nesl_utility/Simulink-PS Converter  PhysicalDomain=network_engine_domain  SubClassName=ps_input  LeftPortType=input  RightPortType=output  PseudoPeriodic=off  Frequencies=[]  NoiseDistribution=none  NoiseParameters=[]  Unit=m^2  AffineConversion=off  FilteringAndDerivatives=zero  SimscapeFilterOrder=1  InputFilterTimeConstant=0.01  UdotUserProvided=1
  A : PMIOPort  Side=Left
  B : PMIOPort  Port=2  Side=Right
  flow : PMIOPort  Port=3  Side=Right
  wires:
  Gain/1 -> m^2/1
  Valve_Commnad/1 -> Gain/1
  connections:
  flow/RConn1 -- Hydraulic Flow Rate Sensor/RConn1
  Hydraulic Flow Rate Sensor/RConn2 -- B/RConn1
  Hydraulic Flow Rate Sensor/LConn1 -- Valve/RConn1
  Valve/LConn1 -- m^2/RConn1
  Valve/LConn2 -- A/RConn1

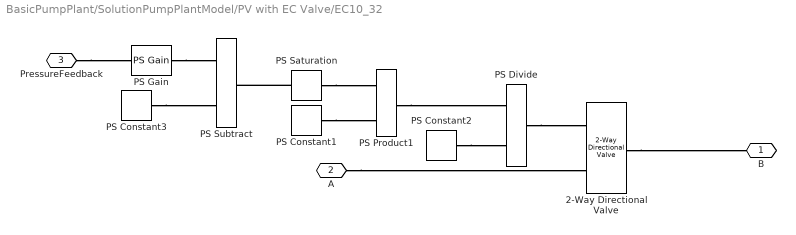
== system BasicPumpPlant/SolutionPumpPlantModel/PV with EC Valve/EC10_32 ==
  2-Way Directional Valve : sh_lib/Valves/Directional Valves/2-Way Directional Valve  mdl_type=2  area_max=0.5e-4 m^2  opening_max=0.005 m  opening_tab=ValveOpeningVector_in in  area_tab=ValvePassageAreaVector_in2 in^2  pressure_tab=[-10000000, -5000000, -2000000, 2000000, 5000000, 10000000] Pa  flow_rate_tab=[-1e-07, -7.0711e-08, -4.4721e-08, 4.4721e-08, 7.0711e-08, 1e-07; -2.0352e-05, -1.4391e-05, -9.1017e-06, 9.1017e-06, 1.4391e-05, 2.0352e-05; -.0040736, -.0028805, -.0018218, .0018218, .0028805, .0040736; -.011438, -.0080879, -.0051152, .0051152, .0080879, .011438; -.034356, -.024293, -.015364, .015364, .024293, .034356] m^3/s  interp_method=1  extrap_method=2  C_d=0.7  x_0=0 m  A_leak=1e-12 m^2  lam_spec=1  B_lam=0.999  Re_cr=12
      settings: InternalSimscapePortConfiguration="{\"Bottom\":[],\"Left\":[{\"id\":\"S\",\"label\":\"S\",\"type\":\"input\"},{\"id\":\"A\",\"label\":\"A\",\"type\":\"foundation.hydraulic.hydraulic\"}],\"Right\":[{\"id\":\"B\",\"label\":\"B\",\"type\":\"foundation.hydraulic.hydraulic\"}],\"Top\":[]}"
  PS Constant1 : fl_lib/Physical Signals/Sources/PS Constant  constant=PistonArea_in2
  PS Constant2 : fl_lib/Physical Signals/Sources/PS Constant  constant=SpringRate_lbfperin
  PS Constant3 : fl_lib/Physical Signals/Sources/PS Constant  constant=PreloadPressure_psi
  PS Divide : fl_ps_legacy_lib/Legacy Physical Signals/Functions/PS Divide
      settings: InternalSimscapePortConfiguration="{\"Bottom\":[],\"Left\":[{\"id\":\"I1\",\"label\":\"\",\"type\":\"input\"},{\"id\":\"I2\",\"label\":\"\",\"type\":\"input\"}],\"Right\":[{\"id\":\"O\",\"label\":\"\",\"type\":\"output\"}],\"Top\":[]}"
  PS Gain : fl_ps_legacy_lib/Legacy Physical Signals/Functions/PS Gain  gain=Pascal_To_psi
  PS Product1 : fl_ps_legacy_lib/Legacy Physical Signals/Functions/PS Product
  PS Saturation : fl_ps_legacy_lib/Legacy Physical Signals/Nonlinear Operators/PS Saturation  upper_limit=inf  lower_limit=0
      settings: InternalSimscapePortConfiguration="{\"Bottom\":[],\"Left\":[{\"id\":\"I\",\"label\":\"\",\"type\":\"input\"}],\"Right\":[{\"id\":\"O\",\"label\":\"\",\"type\":\"output\"}],\"Top\":[]}"
  PS Subtract : fl_ps_legacy_lib/Legacy Physical Signals/Functions/PS Subtract
  B : PMIOPort  Side=Right
  A : PMIOPort  Port=2  Side=Left
  PressureFeedback : PMIOPort  Port=3  Side=Left
  connections:
  2-Way Directional Valve/RConn1 -- B/RConn1
  A/RConn1 -- 2-Way Directional Valve/LConn2
  PS Saturation/LConn1 -- PS Subtract/RConn1
  PS Constant3/RConn1 -- PS Subtract/LConn2
  PressureFeedback/RConn1 -- PS Gain/LConn1
  PS Constant1/RConn1 -- PS Product1/LConn2
  PS Saturation/RConn1 -- PS Product1/LConn1
  PS Divide/RConn1 -- 2-Way Directional Valve/LConn1
  PS Product1/RConn1 -- PS Divide/LConn1
  PS Constant2/RConn1 -- PS Divide/LConn2
  PS Gain/RConn1 -- PS Subtract/LConn1

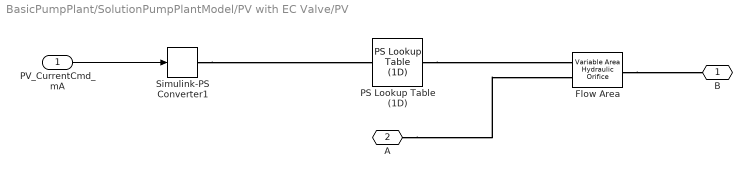
== system BasicPumpPlant/SolutionPumpPlantModel/PV with EC Valve/PV ==
  PV_CurrentCmd_mA : Inport
  Flow Area : fl_lib/Hydraulic/Hydraulic Elements/Variable Area Hydraulic Orifice  C_d=PV_Cd  min_area=1e-12 m^2  lam_spec=2  B_lam=0.999  Re_cr=12  q_specify=off  q_priority=High  q=1 m^3/s  q_nominal_specify=off  q_nominal_unit=m^3/s  q_nominal_value=1  p_specify=off  p_priority=High  p=0 Pa  p_nominal_specify=off  p_nominal_unit=Pa  p_nominal_value=1
      settings: InternalSimscapePortConfiguration="{\"Bottom\":[],\"Left\":[{\"id\":\"AR\",\"label\":\"AR\",\"type\":\"input\"},{\"id\":\"A\",\"label\":\"A\",\"type\":\"foundation.hydraulic.hydraulic\"}],\"Right\":[{\"id\":\"B\",\"label\":\"B\",\"type\":\"foundation.hydraulic.hydraulic\"}],\"Top\":[]}"
  PS Lookup Table (1D) : fl_ps_legacy_lib/Legacy Physical Signals/Lookup Tables/PS Lookup Table (1D)  x=PV_CurrentCmd_mA  f=PV_FlowArea_m2  interp_method=1  extrap_method=1
      settings: InternalSimscapePortConfiguration="{\"Bottom\":[],\"Left\":[{\"id\":\"I\",\"label\":\"x\",\"type\":\"input\"}],\"Right\":[{\"id\":\"O\",\"label\":\"f\",\"type\":\"output\"}],\"Top\":[]}"
  Simulink-PS Converter1 : nesl_utility/Simulink-PS Converter  PhysicalDomain=network_engine_domain  SubClassName=ps_input  LeftPortType=input  RightPortType=output  PseudoPeriodic=off  Frequencies=[]  NoiseDistribution=none  NoiseParameters=[]  Unit=mA  AffineConversion=off  FilteringAndDerivatives=filter  SimscapeFilterOrder=1  InputFilterTimeConstant=0.001  UdotUserProvided=0
  B : PMIOPort  Side=Right
  A : PMIOPort  Port=2  Side=Left
  wires:
  PV_CurrentCmd_mA/1 -> Simulink-PS Converter1/1
  connections:
  PS Lookup Table (1D)/RConn1 -- Flow Area/LConn1
  Simulink-PS Converter1/RConn1 -- PS Lookup Table (1D)/LConn1
  A/RConn1 -- Flow Area/LConn2
  Flow Area/RConn1 -- B/RConn1
